simulink model "ACA_ModelLegoCar_v071"  (R2017b)
settings: Solver=VariableStepAuto  StartTime=0.0  StopTime=20  RelTol=1e-20
PreLoadFcn:
  | InitPar7_1
values from neighbouring files (symbols this model uses):
  CM_Actuator_NonlinarityType = 0    [InitPar7_1.m]
  CM_Actuator_SpeedDependent_MaxGainSpeedOffset = .1    (= 0.1)    [InitPar7_1.m]
  CM_Actuator_SpeedDependent_MinGain = 0.5    [InitPar7_1.m]
  CM_Actuator_SpeedDependent_ZeroSpeedGain = 0.7    [InitPar7_1.m]
  CM_CarWaight = 2    [InitPar7_1.m]
  CM_EnableActuatorQuantizer = 1    [InitPar7_1.m]
  CM_EnableBlockWheel = 1    [InitPar7_1.m]
  CM_EnableWheelSpin = 1    [InitPar7_1.m]
  CM_PWM_FixedOff_offset = 25    [InitPar7_1.m]
  CM_PWM_Type = 1    [InitPar7_1.m]
  CM_RelativeTorqueConstant = 0.0023    [InitPar7_1.m]
  CM_ViscousFriction = 0.018    [InitPar7_1.m]
  CM_WheelInertia = 0.000009    (= 9e-06)    [InitPar7_1.m]
  CM_WheelRadius = 0.03    [InitPar7_1.m]
  CM_WheelSpinInputSlope = 84.5    [InitPar7_1.m]
  CM_WheelSpinInputThresholdStandStill = 70    [InitPar7_1.m]
  FWS_EnableSensor = 0    [InitPar7_1.m]
  GravitinationalAcceleration = 9.82    [InitPar7_1.m]
  MAS_EnablePeriodicErrorAmplitude = 1    [InitPar7_1.m]
  MAS_EnableSensorQuantizer = 1    [InitPar7_1.m]
  MAS_PeriodicErrorAmplitude = 0.7*2*pi/360    (= 0.012217304764)    [InitPar7_1.m]
  One = 1    [InitPar7_1.m]
  Rad2DegFactor = 360/2/pi    (= 57.2957795131)    [InitPar7_1.m]
  USS_EnableError = 1    [InitPar7_1.m]
  USS_EnableSensorQuantizer = 1    [InitPar7_1.m]
  USS_LargeMaxValue = 1    [InitPar7_1.m]
  USS_UnitConversion = 1    [InitPar7_1.m]
libraries: simulink x3
settings Model: Creator=au521529  LastModifiedBy=au521529

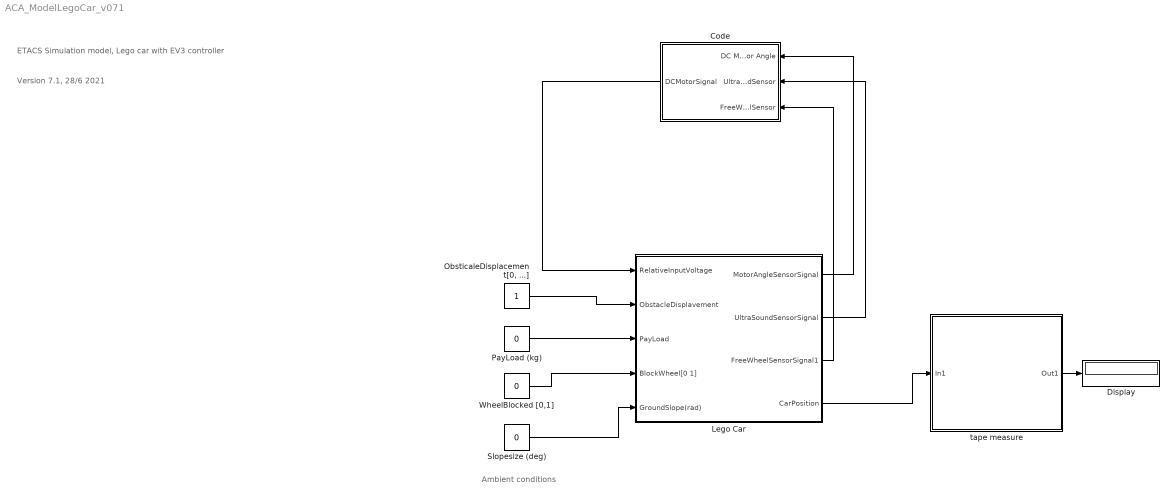
== system ACA_ModelLegoCar_v071 ==
  note: Ambient conditions
  note: Version 7.1, 28/6 2021
  note: ETACS Simulation model, Lego car with EV3 controller
  Code : Subsystem
      mask Display: image('Pic_SimulinkController.jpg');
  Display : Display
      settings: Decimation=2
  Lego Car : Subsystem
      mask DialogControl DescGroupVar Prompt: Logo Car
      mask DialogControl DescTextVar Prompt: This block simulates the mechanical part of the Lego Car. The imput is the scaled DC motor voltage [-100;0;100], where "100" corresponds to the maximum voltage, and "0" corresponds to 0 V. The Lego car has a base waight, driving the no-load dynamics. An additional payload can be applied by teh input port PayLoad (additional waigth in kg).
      mask Display: image(imread('FotoLegoBil.jpg'))
  "ObsticaleDisplacement[0, ...]" : Constant
  PayLoad (kg) : Constant  Value=0
  Slopesize (deg) : Constant  Value=0
  WheelBlocked [0,1] : Constant  Value=0
  tape measure : Subsystem
      mask Display: image('Pic_MaaleBaand.jpg');
  wires:
  Lego Car/1(MotorAngleSensorSignal) -> Code/1(DC Motor Angle)
  Lego Car/2(UltraSoundSensorSignal) -> Code/2(UltraSoundSensor)
  Lego Car/4(CarPosition) -> tape measure/1(In1)
  tape measure/1(Out1) -> Display/1
  Code/1(DCMotorSignal) -> Lego Car/1(RelativeInputVoltage)
  "ObsticaleDisplacement[0, ...]"/1 -> Lego Car/2("ObstacleDisplavement ")
  PayLoad (kg)/1 -> Lego Car/3(PayLoad)
  WheelBlocked [0,1]/1 -> Lego Car/4(BlockWheel[0 1])
  Lego Car/3(FreeWheelSensorSignal1) -> Code/3(FreeWheelSensor)
  Slopesize (deg)/1 -> Lego Car/5(GroundSlope(rad))

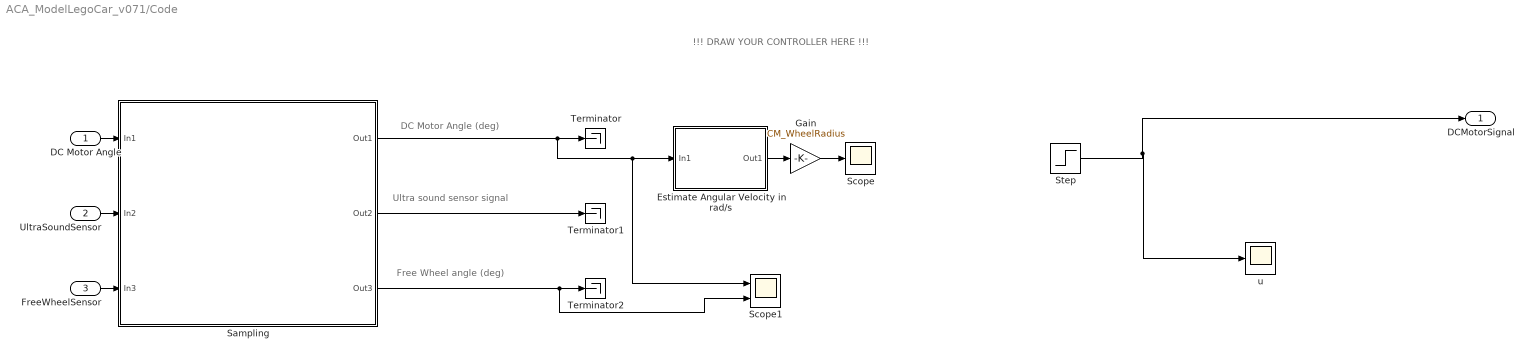
== system ACA_ModelLegoCar_v071/Code ==
  note: Ultra sound sensor signal
  note: Free Wheel angle (deg)
  note: DC Motor Angle (deg)
  note: !!! DRAW YOUR CONTROLLER HERE !!!
  DC Motor Angle : Inport
  UltraSoundSensor : Inport  Port=2
  FreeWheelSensor : Inport  Port=3
  Estimate Angular Velocity in rad/s : Subsystem
  Gain : Gain  Gain=CM_WheelRadius
  Sampling : Subsystem  mask{SystemTs=.01}
      mask prompts: SystemTs "Sampling time in seconds"
      mask DialogControl SystemTs Tooltip: Enter sampling time in seconds
      mask Display: image('Pic_Sampling.jpg');
  Scope : Scope
  Scope1 : Scope  NumInputPorts=2
  Step : Step  After=50  SampleTime=0
  Terminator : Terminator
  Terminator1 : Terminator
  Terminator2 : Terminator
  u : Scope
  DCMotorSignal : Outport
  wires:
  DC Motor Angle/1 -> Sampling/1(In1)
  UltraSoundSensor/1 -> Sampling/2(In2)
  Sampling/1(Out1) -> Scope1/1, Estimate Angular Velocity in rad/s/1(In1), Terminator/1
  Sampling/2(Out2) -> Terminator1/1
  Step/1 -> DCMotorSignal/1, u/1
  Estimate Angular Velocity in rad/s/1(Out1) -> Gain/1
  FreeWheelSensor/1 -> Sampling/3(In3)
  Sampling/3(Out3) -> Scope1/2, Terminator2/1
  Gain/1 -> Scope/1

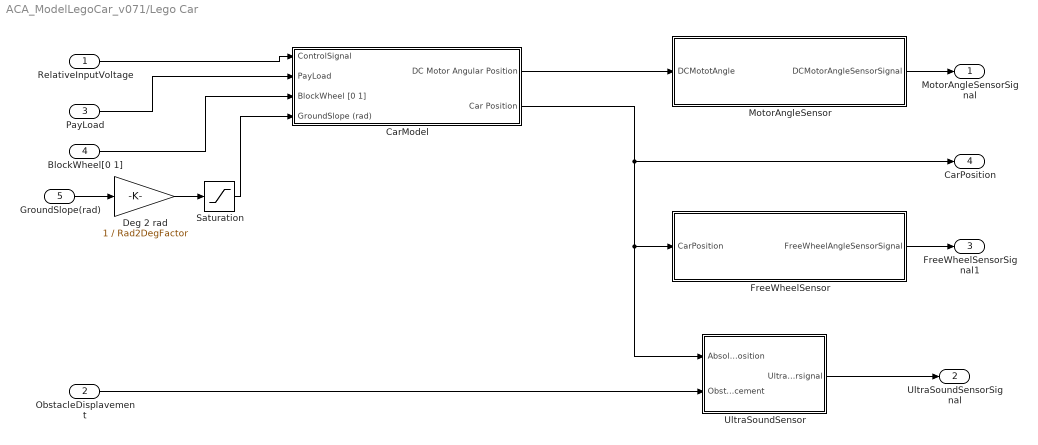
== system ACA_ModelLegoCar_v071/Lego Car ==
  RelativeInputVoltage : Inport
  "ObstacleDisplavement " : Inport  Port=2
  PayLoad : Inport  Port=3
  BlockWheel[0 1] : Inport  Port=4
  GroundSlope(rad) : Inport  Port=5
  CarModel : Subsystem
  Deg 2 rad : Gain  Gain=1 / Rad2DegFactor
  FreeWheelSensor : Subsystem
  MotorAngleSensor : Subsystem
  Saturation : Saturate  UpperLimit=pi/2*.99  LowerLimit=-pi/2*.99
  UltraSoundSensor : Subsystem
  MotorAngleSensorSignal : Outport
  UltraSoundSensorSignal : Outport  Port=2
  FreeWheelSensorSignal1 : Outport  Port=3
  CarPosition : Outport  Port=4
  wires:
  RelativeInputVoltage/1 -> CarModel/1(ControlSignal)
  "ObstacleDisplavement "/1 -> UltraSoundSensor/2(ObstacleDisplacement)
  UltraSoundSensor/1(UltraSoundSensorsignal) -> UltraSoundSensorSignal/1
  MotorAngleSensor/1(DCMotorAngleSensorSignal) -> MotorAngleSensorSignal/1
  CarModel/1(DC Motor Angular Position) -> MotorAngleSensor/1(DCMototAngle)
  PayLoad/1 -> CarModel/2(PayLoad)
  BlockWheel[0 1]/1 -> CarModel/3(BlockWheel [0 1])
  CarModel/2(Car Position) -> FreeWheelSensor/1(CarPosition), UltraSoundSensor/1(AbsoluteCarPosition), CarPosition/1
  FreeWheelSensor/1(FreeWheelAngleSensorSignal) -> FreeWheelSensorSignal1/1
  GroundSlope(rad)/1 -> Deg 2 rad/1
  Deg 2 rad/1 -> Saturation/1
  Saturation/1 -> CarModel/4(GroundSlope (rad))

== system ACA_ModelLegoCar_v071/tape measure ==
  In1 : Inport
  Gain : Gain  Gain=100
  Out1 : Outport
  wires:
  In1/1 -> Gain/1
  Gain/1 -> Out1/1

== system ACA_ModelLegoCar_v071/Code/Estimate Angular Velocity in rad//s ==
  In1 : Inport
  1/Ts : Gain  Gain=1/.01
  Sum : Sum  Inputs=|+-
  Unit Delay : UnitDelay  SampleTime=-1
  deg2rad : Gain  Gain=2*pi/360
  Out1 : Outport
  wires:
  Unit Delay/1 -> Sum/2
  In1/1 -> deg2rad/1
  deg2rad/1 -> Unit Delay/1, Sum/1
  1/Ts/1 -> Out1/1
  Sum/1 -> 1/Ts/1

== system ACA_ModelLegoCar_v071/Code/Sampling ==
  note: !!! DRAW YOUR CONTROLLER HERE !!!
  In1 : Inport
  In2 : Inport  Port=2
  In3 : Inport  Port=3
  Zero-Order Hold1 : ZeroOrderHold  SampleTime=SystemTs
  Zero-Order Hold2 : ZeroOrderHold  SampleTime=SystemTs
  Zero-Order Hold3 : ZeroOrderHold  SampleTime=SystemTs
  Out1 : Outport
  Out2 : Outport  Port=2
  Out3 : Outport  Port=3
  wires:
  In1/1 -> Zero-Order Hold2/1
  In2/1 -> Zero-Order Hold1/1
  Zero-Order Hold1/1 -> Out2/1
  Zero-Order Hold2/1 -> Out1/1
  Zero-Order Hold3/1 -> Out3/1
  In3/1 -> Zero-Order Hold3/1

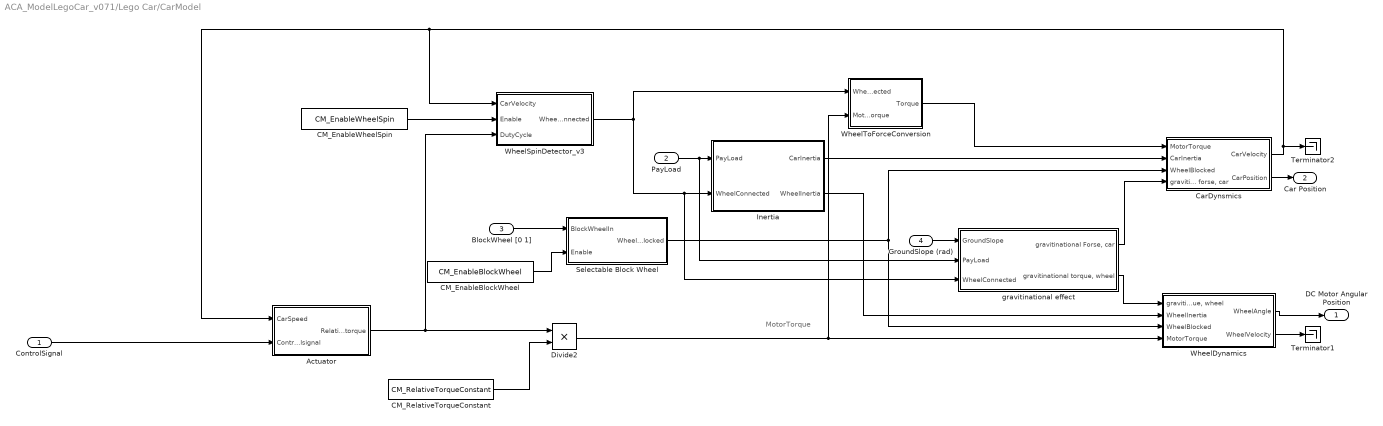
== system ACA_ModelLegoCar_v071/Lego Car/CarModel ==
  note: MotorTorque
  ControlSignal : Inport
  PayLoad : Inport  Port=2
  BlockWheel [0 1] : Inport  Port=3
  GroundSlope (rad) : Inport  Port=4
  Actuator : Subsystem
  CM_EnableBlockWheel : Constant  Value=CM_EnableBlockWheel
  CM_EnableWheelSpin : Constant  Value=CM_EnableWheelSpin
  CM_RelativeTorqueConstant : Constant  Value=CM_RelativeTorqueConstant
  CarDynsmics : Subsystem
  Divide2 : Product  Inputs=**
  Inertia : Subsystem
  Selectable Block Wheel : Subsystem
  Terminator1 : Terminator
  Terminator2 : Terminator
  WheelDynamics : Subsystem
  WheelSpinDetector_v3 : Subsystem
  WheelToForceConversion : Subsystem
  gravitinational effect : Subsystem
  DC Motor Angular Position : Outport
  Car Position : Outport  Port=2
  wires:
  Divide2/1 -> WheelToForceConversion/2(MotorTorque), WheelDynamics/4(MotorTorque)
  CM_RelativeTorqueConstant/1 -> Divide2/2
  PayLoad/1 -> gravitinational effect/2(PayLoad), Inertia/1(PayLoad)
  CM_EnableBlockWheel/1 -> Selectable Block Wheel/2(Enable)
  BlockWheel [0 1]/1 -> Selectable Block Wheel/1(BlockWheelIn)
  CM_EnableWheelSpin/1 -> WheelSpinDetector_v3/2(Enable)
  WheelToForceConversion/1(Torque) -> CarDynsmics/1(MotorTorque)
  Inertia/1(CarInertia) -> CarDynsmics/2(CarInertia)
  CarDynsmics/2(CarPosition) -> Car Position/1
  Inertia/2(WheelInertia) -> WheelDynamics/2(WheelInertia)
  WheelDynamics/1(WheelAngle) -> DC Motor Angular Position/1
  Selectable Block Wheel/1(WheelBlocked) -> WheelDynamics/3(WheelBlocked), CarDynsmics/3(WheelBlocked)
  WheelDynamics/2(WheelVelocity) -> Terminator1/1
  WheelSpinDetector_v3/1(WheelConnected) -> gravitinational effect/3(WheelConnected), Inertia/2(WheelConnected), WheelToForceConversion/1(WheelConnected)
  CarDynsmics/1(CarVelocity) -> Terminator2/1, Actuator/1(CarSpeed), WheelSpinDetector_v3/1(CarVelocity)
  Actuator/1(Relativetorque) -> Divide2/1, WheelSpinDetector_v3/3(DutyCycle)
  ControlSignal/1 -> Actuator/2(Controlsignal)
  gravitinational effect/2("gravitinational torque, wheel") -> WheelDynamics/1("gravitinational torque, wheel")
  gravitinational effect/1("gravitinational Forse, car") -> CarDynsmics/4("gravitinational forse, car")
  GroundSlope (rad)/1 -> gravitinational effect/1(GroundSlope)

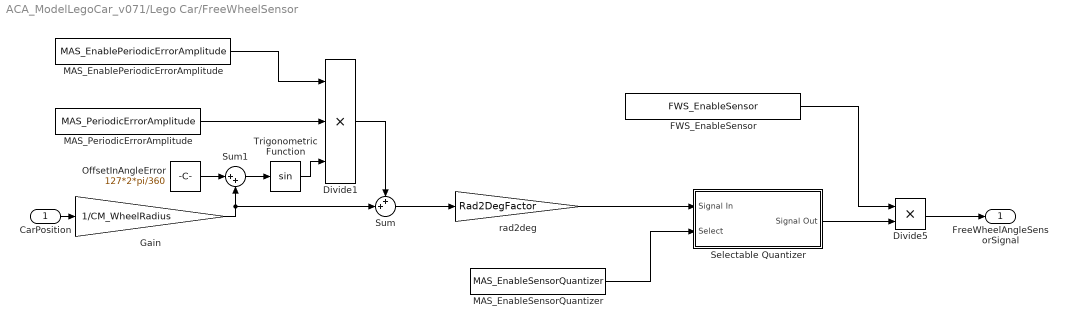
== system ACA_ModelLegoCar_v071/Lego Car/FreeWheelSensor ==
  CarPosition : Inport
  Divide1 : Product  Inputs=***
  Divide5 : Product  Inputs=**
  FWS_EnableSensor : Constant  Value=FWS_EnableSensor
  Gain : Gain  Gain=1/CM_WheelRadius
  MAS_EnablePeriodicErrorAmplitude : Constant  Value=MAS_EnablePeriodicErrorAmplitude
  MAS_EnableSensorQuantizer : Constant  Value=MAS_EnableSensorQuantizer
  MAS_PeriodicErrorAmplitude : Constant  Value=MAS_PeriodicErrorAmplitude
  OffsetInAngleError : Constant  Value=127*2*pi/360
  Selectable Quantizer : Subsystem
  Sum : Sum  Inputs=++|
  Sum1 : Sum  Inputs=|++
  Trigonometric Function : Trigonometry
  rad2deg : Gain  Gain=Rad2DegFactor
  FreeWheelAngleSensorSignal : Outport
  wires:
  Divide1/1 -> Sum/1
  Sum/1 -> rad2deg/1
  rad2deg/1 -> Selectable Quantizer/1(Signal In)
  MAS_EnableSensorQuantizer/1 -> Selectable Quantizer/2(Select)
  Trigonometric Function/1 -> Divide1/3
  MAS_PeriodicErrorAmplitude/1 -> Divide1/2
  MAS_EnablePeriodicErrorAmplitude/1 -> Divide1/1
  Sum1/1 -> Trigonometric Function/1
  OffsetInAngleError/1 -> Sum1/1
  Gain/1 -> Sum/2, Sum1/2
  CarPosition/1 -> Gain/1
  Selectable Quantizer/1(Signal Out) -> Divide5/2
  Divide5/1 -> FreeWheelAngleSensorSignal/1
  FWS_EnableSensor/1 -> Divide5/1

== system ACA_ModelLegoCar_v071/Lego Car/MotorAngleSensor ==
  DCMototAngle : Inport
  Divide1 : Product  Inputs=***
  MAS_EnablePeriodicErrorAmplitude : Constant  Value=MAS_EnablePeriodicErrorAmplitude
  MAS_EnableSensorQuantizer : Constant  Value=MAS_EnableSensorQuantizer
  MAS_PeriodicErrorAmplitude : Constant  Value=MAS_PeriodicErrorAmplitude
  Selectable Quantizer : Subsystem
  Sum : Sum  Inputs=++|
  Trigonometric Function : Trigonometry
  rad2deg : Gain  Gain=Rad2DegFactor
  DCMotorAngleSensorSignal : Outport
  wires:
  Divide1/1 -> Sum/1
  DCMototAngle/1 -> Trigonometric Function/1, Sum/2
  Sum/1 -> rad2deg/1
  rad2deg/1 -> Selectable Quantizer/1(Signal In)
  MAS_EnableSensorQuantizer/1 -> Selectable Quantizer/2(Select)
  Trigonometric Function/1 -> Divide1/3
  MAS_PeriodicErrorAmplitude/1 -> Divide1/2
  MAS_EnablePeriodicErrorAmplitude/1 -> Divide1/1
  Selectable Quantizer/1(Signal Out) -> DCMotorAngleSensorSignal/1

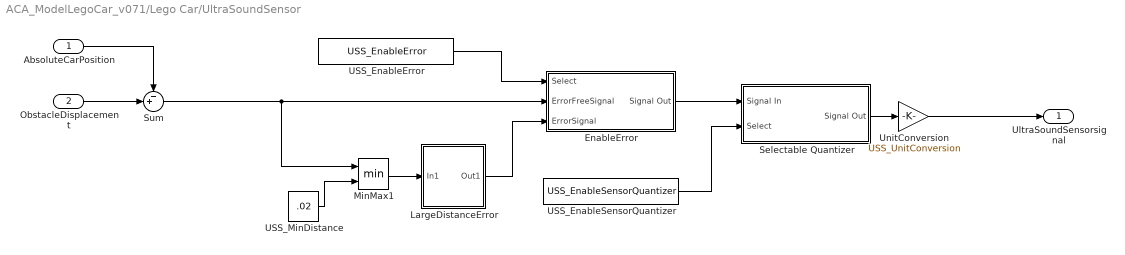
== system ACA_ModelLegoCar_v071/Lego Car/UltraSoundSensor ==
  AbsoluteCarPosition : Inport
  ObstacleDisplacement : Inport  Port=2
  EnableError : Subsystem
  LargeDistanceError : Subsystem
  MinMax1 : MinMax  Inputs=2
  Selectable Quantizer : Subsystem
  Sum : Sum  Inputs=-+|
  USS_EnableError : Constant  Value=USS_EnableError
  USS_EnableSensorQuantizer : Constant  Value=USS_EnableSensorQuantizer
  USS_MinDistance : Constant  Value=.02
  UnitConversion : Gain  Gain=USS_UnitConversion
  UltraSoundSensorsignal : Outport
  wires:
  ObstacleDisplacement/1 -> Sum/2
  AbsoluteCarPosition/1 -> Sum/1
  USS_MinDistance/1 -> MinMax1/2
  Sum/1 -> EnableError/2(ErrorFreeSignal), MinMax1/1
  LargeDistanceError/1(Out1) -> EnableError/3(ErrorSignal)
  MinMax1/1 -> LargeDistanceError/1(In1)
  Selectable Quantizer/1(Signal Out) -> UnitConversion/1
  USS_EnableSensorQuantizer/1 -> Selectable Quantizer/2(Select)
  EnableError/1(Signal Out) -> Selectable Quantizer/1(Signal In)
  USS_EnableError/1 -> EnableError/1(Select)
  UnitConversion/1 -> UltraSoundSensorsignal/1

== system ACA_ModelLegoCar_v071/Lego Car/CarModel/Actuator ==
  note: Duty sycle
  CarSpeed : Inport
  Controlsignal : Inport  Port=2
  ActuatorNonlinarity : Subsystem
  CM_Actuator_NonlinarityType : Constant  Value=CM_Actuator_NonlinarityType
  CM_PWM_Type : Constant  Value=CM_PWM_Type
  CM_RelativeTorqueConstant1 : Constant  Value=CM_EnableActuatorQuantizer
  PWM and communication : Subsystem
  Relativetorque : Outport
  wires:
  PWM and communication/1(DutyScycle(procentage)) -> ActuatorNonlinarity/2(ControlSignal)
  CM_RelativeTorqueConstant1/1 -> PWM and communication/2(EnableQuantizer)
  CM_Actuator_NonlinarityType/1 -> ActuatorNonlinarity/3(NonlinarityType [0 1])
  CM_PWM_Type/1 -> PWM and communication/3(Select_PWM_type)
  ActuatorNonlinarity/1(DutyScycle(procentage)) -> Relativetorque/1
  Controlsignal/1 -> PWM and communication/1(ControlSignal)
  CarSpeed/1 -> ActuatorNonlinarity/1(CarSpeed)

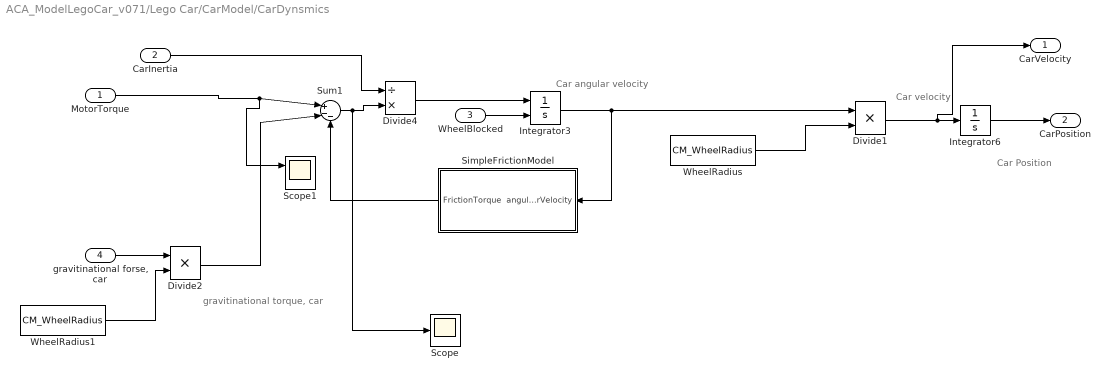
== system ACA_ModelLegoCar_v071/Lego Car/CarModel/CarDynsmics ==
  note: gravitinational torque, car
  note: Car velocity
  note: Car angular velocity
  note: Car Position
  MotorTorque : Inport
  CarInertia : Inport  Port=2
  WheelBlocked : Inport  Port=3
  "gravitinational forse, car" : Inport  Port=4
  Divide1 : Product  Inputs=**
  Divide2 : Product  Inputs=**
  Divide4 : Product  Inputs=/*
  Integrator3 : Integrator  ExternalReset=level
  Integrator6 : Integrator
  Scope : Scope
  Scope1 : Scope  NumInputPorts=2
  SimpleFrictionModel : Subsystem
  Sum1 : Sum  Inputs=|+--
  WheelRadius : Constant  Value=CM_WheelRadius
  WheelRadius1 : Constant  Value=CM_WheelRadius
  CarVelocity : Outport
  CarPosition : Outport  Port=2
  wires:
  Divide4/1 -> Integrator3/1
  Sum1/1 -> Scope/1, Divide4/2
  Integrator3/1 -> Divide1/1, SimpleFrictionModel/1(angularVelocity)
  Integrator6/1 -> CarPosition/1
  WheelBlocked/1 -> Integrator3/2
  SimpleFrictionModel/1(FrictionTorque) -> Sum1/3
  Divide1/1 -> CarVelocity/1, Integrator6/1
  WheelRadius/1 -> Divide1/2
  "gravitinational forse, car"/1 -> Divide2/1
  WheelRadius1/1 -> Divide2/2
  MotorTorque/1 -> Scope1/1, Sum1/1
  CarInertia/1 -> Divide4/1
  Divide2/1 -> Sum1/2

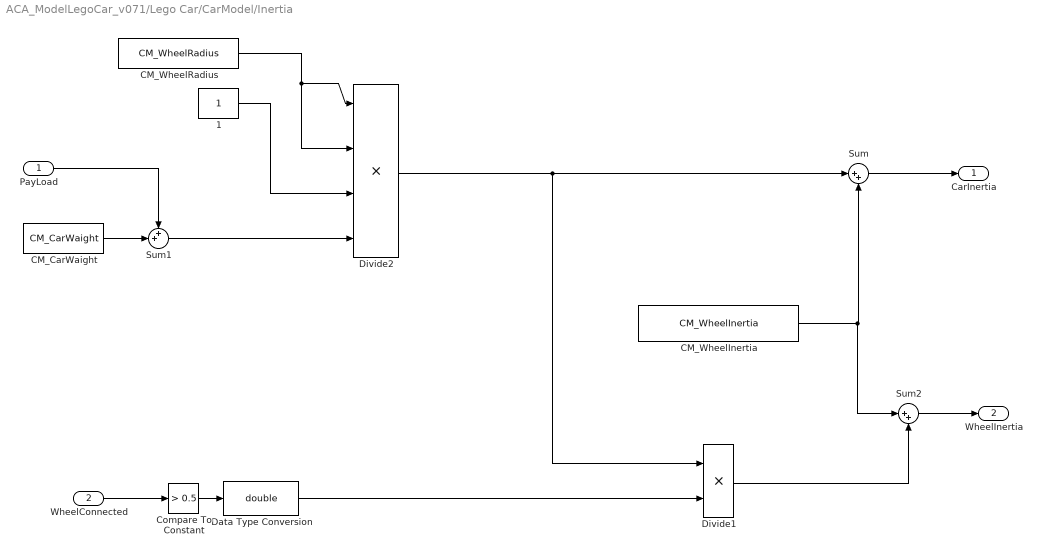
== system ACA_ModelLegoCar_v071/Lego Car/CarModel/Inertia ==
  PayLoad : Inport
  WheelConnected : Inport  Port=2
  "1 " : Constant
  CM_CarWaight : Constant  Value=CM_CarWaight
  CM_WheelInertia : Constant  Value=CM_WheelInertia
  CM_WheelRadius : Constant  Value=CM_WheelRadius
  Compare To Constant : simulink/Logic and Bit Operations/Compare To Constant  relop=>  const=0.5  OutDataTypeStr=boolean
  Data Type Conversion : DataTypeConversion  OutDataTypeStr=double
  Divide1 : Product  Inputs=**
  Divide2 : Product  Inputs=****
  Sum : Sum  Inputs=|++
  Sum1 : Sum  Inputs=++|
  Sum2 : Sum  Inputs=|++
  CarInertia : Outport
  WheelInertia : Outport  Port=2
  wires:
  CM_WheelRadius/1 -> Divide2/1, Divide2/2
  PayLoad/1 -> Sum1/1
  "1 "/1 -> Divide2/3
  CM_CarWaight/1 -> Sum1/2
  Sum1/1 -> Divide2/4
  Divide2/1 -> Divide1/1, Sum/1
  Sum/1 -> CarInertia/1
  CM_WheelInertia/1 -> Sum2/1, Sum/2
  Data Type Conversion/1 -> Divide1/2
  Compare To Constant/1 -> Data Type Conversion/1
  WheelConnected/1 -> Compare To Constant/1
  Divide1/1 -> Sum2/2
  Sum2/1 -> WheelInertia/1

== system ACA_ModelLegoCar_v071/Lego Car/CarModel/Selectable Block Wheel ==
  BlockWheelIn : Inport
  Enable : Inport  Port=2
  Compare To Constant : simulink/Logic and Bit Operations/Compare To Constant  relop=>  const=0.5  OutDataTypeStr=boolean
  Data Type Conversion : DataTypeConversion  OutDataTypeStr=double
  Divide4 : Product  Inputs=**
  WheelBlocked : Outport
  wires:
  Divide4/1 -> WheelBlocked/1
  Enable/1 -> Divide4/2
  Compare To Constant/1 -> Data Type Conversion/1
  Data Type Conversion/1 -> Divide4/1
  BlockWheelIn/1 -> Compare To Constant/1

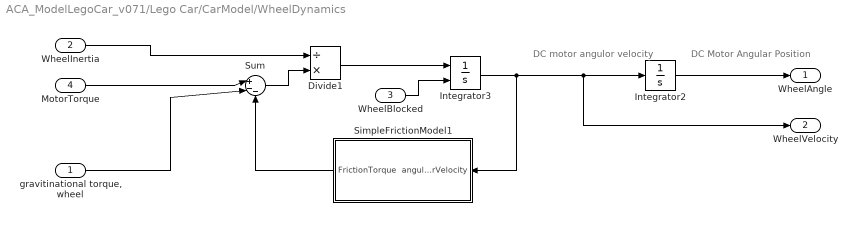
== system ACA_ModelLegoCar_v071/Lego Car/CarModel/WheelDynamics ==
  note: DC Motor Angular Position
  note: DC motor angulor velocity
  "gravitinational torque, wheel" : Inport
  WheelInertia : Inport  Port=2
  WheelBlocked : Inport  Port=3
  MotorTorque : Inport  Port=4
  Divide1 : Product  Inputs=/*
  Integrator2 : Integrator
  Integrator3 : Integrator  ExternalReset=level
  SimpleFrictionModel1 : Subsystem
  Sum : Sum  Inputs=|+--
  WheelAngle : Outport
  WheelVelocity : Outport  Port=2
  wires:
  Integrator2/1 -> WheelAngle/1
  Sum/1 -> Divide1/2
  WheelInertia/1 -> Divide1/1
  MotorTorque/1 -> Sum/1
  Integrator3/1 -> WheelVelocity/1, Integrator2/1, SimpleFrictionModel1/1(angularVelocity)
  Divide1/1 -> Integrator3/1
  WheelBlocked/1 -> Integrator3/2
  SimpleFrictionModel1/1(FrictionTorque) -> Sum/3
  "gravitinational torque, wheel"/1 -> Sum/2

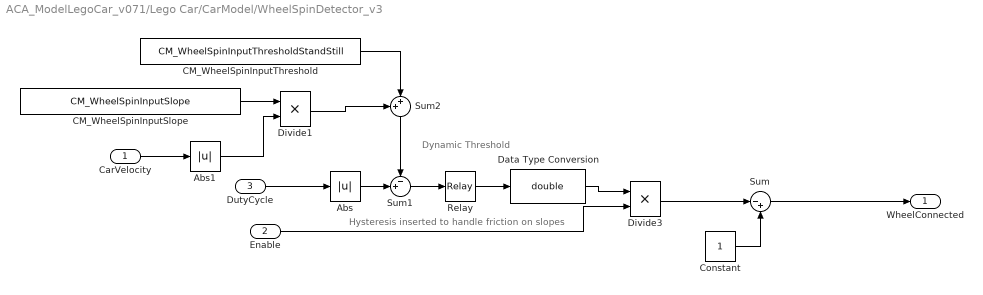
== system ACA_ModelLegoCar_v071/Lego Car/CarModel/WheelSpinDetector_v3 ==
  note: Hysteresis inserted to handle friction on slopes
  note: Dynamic Threshold
  CarVelocity : Inport
  Enable : Inport  Port=2
  DutyCycle : Inport  Port=3
  Abs : Abs
  Abs1 : Abs
  CM_WheelSpinInputSlope : Constant  Value=CM_WheelSpinInputSlope
  CM_WheelSpinInputThreshold : Constant  Value=CM_WheelSpinInputThresholdStandStill
  Constant : Constant
  Data Type Conversion : DataTypeConversion  OutDataTypeStr=double
  Divide1 : Product  Inputs=**
  Divide3 : Product  Inputs=**
  Relay : Relay  OnSwitchValue=.01  OffSwitchValue=.001
  Sum : Sum  Inputs=|-+
  Sum1 : Sum  Inputs=-+|
  Sum2 : Sum  Inputs=++|
  WheelConnected : Outport
  wires:
  Data Type Conversion/1 -> Divide3/1
  Relay/1 -> Data Type Conversion/1
  DutyCycle/1 -> Abs/1
  Enable/1 -> Divide3/2
  Constant/1 -> Sum/2
  Divide3/1 -> Sum/1
  Abs/1 -> Sum1/2
  Sum1/1 -> Relay/1
  CM_WheelSpinInputThreshold/1 -> Sum2/2
  Sum2/1 -> Sum1/1
  Divide1/1 -> Sum2/1
  CM_WheelSpinInputSlope/1 -> Divide1/1
  CarVelocity/1 -> Abs1/1
  Abs1/1 -> Divide1/2
  Sum/1 -> WheelConnected/1

== system ACA_ModelLegoCar_v071/Lego Car/CarModel/WheelToForceConversion ==
  WheelConnected : Inport
  MotorTorque : Inport  Port=2
  1 : Constant
  Divide6 : Product  Inputs=***
  Scope : Scope
  Torque : Outport
  wires:
  WheelConnected/1 -> Divide6/2
  1/1 -> Divide6/1
  Divide6/1 -> Scope/1, Torque/1
  MotorTorque/1 -> Divide6/3

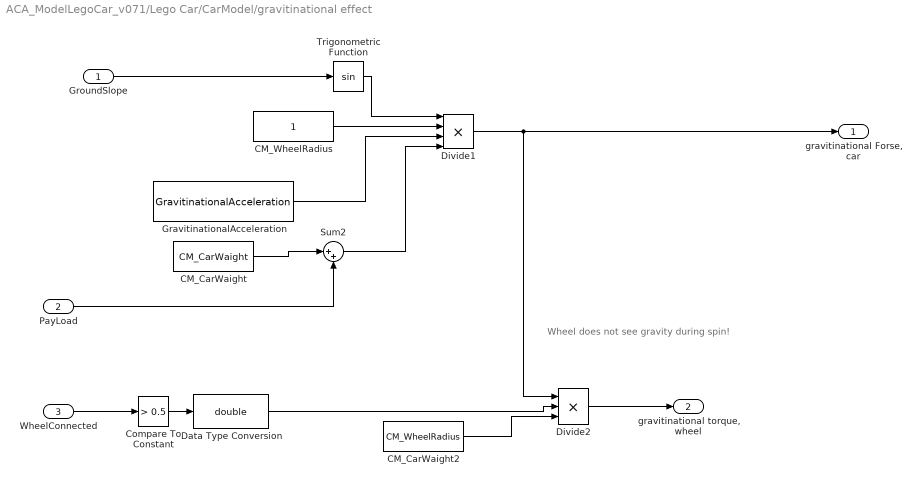
== system ACA_ModelLegoCar_v071/Lego Car/CarModel/gravitinational effect ==
  note: Wheel does not see gravity during spin!
  GroundSlope : Inport
  PayLoad : Inport  Port=2
  WheelConnected : Inport  Port=3
  CM_CarWaight : Constant  Value=CM_CarWaight
  CM_CarWaight2 : Constant  Value=CM_WheelRadius
  "CM_WheelRadius " : Constant
  Compare To Constant : simulink/Logic and Bit Operations/Compare To Constant  relop=>  const=0.5  OutDataTypeStr=boolean
  Data Type Conversion : DataTypeConversion  OutDataTypeStr=double
  Divide1 : Product  Inputs=****
  Divide2 : Product  Inputs=***
  GravitinationalAcceleration : Constant  Value=GravitinationalAcceleration
  Sum2 : Sum  Inputs=|++
  Trigonometric Function : Trigonometry
  "gravitinational Forse, car" : Outport
  "gravitinational torque, wheel" : Outport  Port=2
  wires:
  PayLoad/1 -> Sum2/2
  Trigonometric Function/1 -> Divide1/1
  Sum2/1 -> Divide1/4
  "CM_WheelRadius "/1 -> Divide1/2
  GravitinationalAcceleration/1 -> Divide1/3
  CM_CarWaight/1 -> Sum2/1
  GroundSlope/1 -> Trigonometric Function/1
  WheelConnected/1 -> Compare To Constant/1
  Compare To Constant/1 -> Data Type Conversion/1
  Data Type Conversion/1 -> Divide2/2
  Divide2/1 -> "gravitinational torque, wheel"/1
  CM_CarWaight2/1 -> Divide2/3
  Divide1/1 -> "gravitinational Forse, car"/1, Divide2/1

== system ACA_ModelLegoCar_v071/Lego Car/FreeWheelSensor/Selectable Quantizer ==
  Signal In : Inport
  Select : Inport  Port=2
  Divide4 : Product  Inputs=**
  Divide5 : Product  Inputs=**
  One : Constant
  Quantizer : Quantizer  QuantizationInterval=1
  Sum1 : Sum  Inputs=-+|
  Sum2 : Sum  Inputs=+|+
  Signal Out : Outport
  wires:
  Sum2/1 -> Signal Out/1
  Quantizer/1 -> Divide5/1
  Signal In/1 -> Divide4/2, Quantizer/1
  Sum1/1 -> Divide4/1
  Select/1 -> Sum1/1, Divide5/2
  Divide4/1 -> Sum2/2
  One/1 -> Sum1/2
  Divide5/1 -> Sum2/1

== system ACA_ModelLegoCar_v071/Lego Car/MotorAngleSensor/Selectable Quantizer ==
  Signal In : Inport
  Select : Inport  Port=2
  Divide4 : Product  Inputs=**
  Divide5 : Product  Inputs=**
  One : Constant
  Quantizer : Quantizer  QuantizationInterval=1
  Sum1 : Sum  Inputs=-+|
  Sum2 : Sum  Inputs=+|+
  Signal Out : Outport
  wires:
  Sum2/1 -> Signal Out/1
  Quantizer/1 -> Divide5/1
  Signal In/1 -> Divide4/2, Quantizer/1
  Sum1/1 -> Divide4/1
  Select/1 -> Sum1/1, Divide5/2
  Divide4/1 -> Sum2/2
  One/1 -> Sum1/2
  Divide5/1 -> Sum2/1

== system ACA_ModelLegoCar_v071/Lego Car/UltraSoundSensor/EnableError ==
  Select : Inport
  ErrorFreeSignal : Inport  Port=2
  ErrorSignal : Inport  Port=3
  Divide4 : Product  Inputs=**
  Divide5 : Product  Inputs=**
  One : Constant  Value=One
  Sum1 : Sum  Inputs=-+|
  Sum2 : Sum  Inputs=+|+
  Signal Out : Outport
  wires:
  Sum2/1 -> Signal Out/1
  ErrorSignal/1 -> Divide5/1
  Sum1/1 -> Divide4/1
  Select/1 -> Sum1/1, Divide5/2
  Divide4/1 -> Sum2/2
  One/1 -> Sum1/2
  Divide5/1 -> Sum2/1
  ErrorFreeSignal/1 -> Divide4/2

== system ACA_ModelLegoCar_v071/Lego Car/UltraSoundSensor/LargeDistanceError ==
  In1 : Inport
  1 : Constant
  Divide : Product  Inputs=/*
  Divide1 : Product  Inputs=**
  Gain : Gain  Gain=-1
  Math Function : Math  SaturateOnIntegerOverflow=on
  MinMax1 : MinMax  Inputs=2
  Sum1 : Sum  Inputs=-+|
  USS_LargeErrorSlope : Constant  Value=.7
  USS_LargeMaxValue : Constant  Value=USS_LargeMaxValue
  Out1 : Outport
  wires:
  Math Function/1 -> Sum1/1
  Sum1/1 -> Divide1/1
  USS_LargeMaxValue/1 -> Divide1/2
  Gain/1 -> Divide/1
  USS_LargeErrorSlope/1 -> Gain/1
  Divide/1 -> Math Function/1
  In1/1 -> MinMax1/2, Divide/2
  1/1 -> Sum1/2
  Divide1/1 -> MinMax1/1
  MinMax1/1 -> Out1/1

== system ACA_ModelLegoCar_v071/Lego Car/UltraSoundSensor/Selectable Quantizer ==
  Signal In : Inport
  Select : Inport  Port=2
  Divide4 : Product  Inputs=**
  Divide5 : Product  Inputs=**
  One : Constant
  Quantizer : Quantizer  QuantizationInterval=1
  Sum1 : Sum  Inputs=-+|
  Sum2 : Sum  Inputs=+|+
  Signal Out : Outport
  wires:
  Sum2/1 -> Signal Out/1
  Quantizer/1 -> Divide5/1
  Signal In/1 -> Divide4/2, Quantizer/1
  Sum1/1 -> Divide4/1
  Select/1 -> Sum1/1, Divide5/2
  Divide4/1 -> Sum2/2
  One/1 -> Sum1/2
  Divide5/1 -> Sum2/1

== system ACA_ModelLegoCar_v071/Lego Car/CarModel/Actuator/ActuatorNonlinarity ==
  note: Constant period PWM
  CarSpeed : Inport
  ControlSignal : Inport  Port=2
  NonlinarityType [0 1] : Inport  Port=3
  Abs1 : Abs
  Divide3 : Product  Inputs=**
  Index Vector : MultiPortSwitch  DataPortOrder=Zero-based contiguous  Inputs=2
  Saturation : Saturate  UpperLimit=1  LowerLimit=0
  Tytpe 1: Polonium : Subsystem
  DutyScycle(procentage) : Outport
  wires:
  ControlSignal/1 -> Divide3/1, Index Vector/2
  Saturation/1 -> Index Vector/1
  Index Vector/1 -> DutyScycle(procentage)/1
  NonlinarityType [0 1]/1 -> Saturation/1
  CarSpeed/1 -> Abs1/1
  Divide3/1 -> Index Vector/3
  Abs1/1 -> Tytpe 1: Polonium/1(In1)
  Tytpe 1: Polonium/1(Out1) -> Divide3/2

== system ACA_ModelLegoCar_v071/Lego Car/CarModel/Actuator/PWM and communication ==
  ControlSignal : Inport
  EnableQuantizer : Inport  Port=2
  Select_PWM_type : Inport  Port=3
  PWM : Subsystem
  Saturation : Saturate  UpperLimit=100  LowerLimit=-100
  Selectable Quantizer : Subsystem
  DutyScycle(procentage) : Outport
  wires:
  ControlSignal/1 -> Saturation/1
  EnableQuantizer/1 -> Selectable Quantizer/2(Enable)
  Select_PWM_type/1 -> PWM/2(PWM_ Type [1 2])
  Selectable Quantizer/1(Signal Out) -> PWM/1(ControlSignal)
  PWM/1(DutyScycle(procentage)) -> DutyScycle(procentage)/1
  Saturation/1 -> Selectable Quantizer/1(Signal In)

== system ACA_ModelLegoCar_v071/Lego Car/CarModel/CarDynsmics/SimpleFrictionModel ==
  angularVelocity : Inport
  CM_ViscousFriction : Constant  Value=CM_ViscousFriction
  Divide4 : Product  Inputs=**
  FrictionTorque : Outport
  wires:
  angularVelocity/1 -> Divide4/2
  CM_ViscousFriction/1 -> Divide4/1
  Divide4/1 -> FrictionTorque/1

== system ACA_ModelLegoCar_v071/Lego Car/CarModel/WheelDynamics/SimpleFrictionModel1 ==
  angularVelocity : Inport
  CM_ViscousFriction : Constant  Value=CM_ViscousFriction
  Divide4 : Product  Inputs=**
  FrictionTorque : Outport
  wires:
  angularVelocity/1 -> Divide4/2
  CM_ViscousFriction/1 -> Divide4/1
  Divide4/1 -> FrictionTorque/1

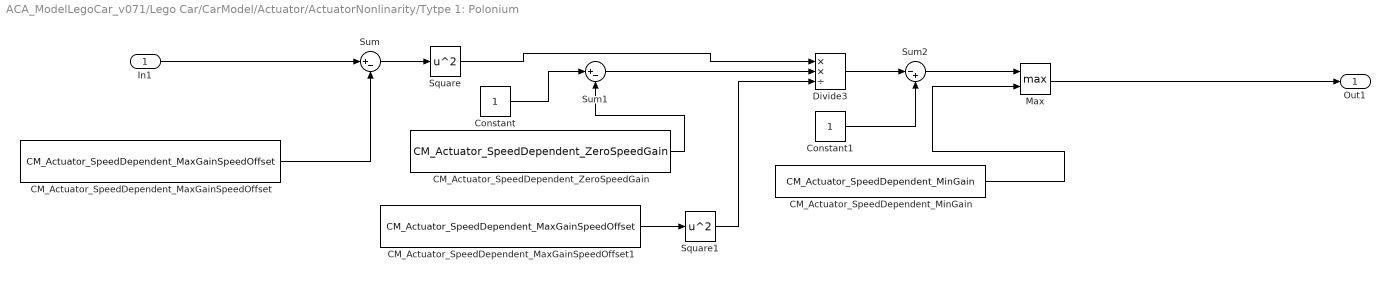
== system ACA_ModelLegoCar_v071/Lego Car/CarModel/Actuator/ActuatorNonlinarity/Tytpe 1: Polonium ==
  In1 : Inport
  CM_Actuator_SpeedDependent_MaxGainSpeedOffset : Constant  Value=CM_Actuator_SpeedDependent_MaxGainSpeedOffset
  CM_Actuator_SpeedDependent_MaxGainSpeedOffset1 : Constant  Value=CM_Actuator_SpeedDependent_MaxGainSpeedOffset
  CM_Actuator_SpeedDependent_MinGain : Constant  Value=CM_Actuator_SpeedDependent_MinGain
  CM_Actuator_SpeedDependent_ZeroSpeedGain : Constant  Value=CM_Actuator_SpeedDependent_ZeroSpeedGain
  Constant : Constant
  Constant1 : Constant
  Divide3 : Product  Inputs=**/
  Max : MinMax  Function=max  Inputs=2
  Square : Math  Operator=square  RndMeth=Zero  SaturateOnIntegerOverflow=on
  Square1 : Math  Operator=square  RndMeth=Zero  SaturateOnIntegerOverflow=on
  Sum : Sum  Inputs=|+-
  Sum1 : Sum  Inputs=|+-
  Sum2 : Sum  Inputs=|-+
  Out1 : Outport
  wires:
  In1/1 -> Sum/1
  Sum/1 -> Square/1
  CM_Actuator_SpeedDependent_MaxGainSpeedOffset/1 -> Sum/2
  Square1/1 -> Divide3/3
  Constant1/1 -> Sum2/2
  Constant/1 -> Sum1/1
  Sum2/1 -> Max/1
  Max/1 -> Out1/1
  Square/1 -> Divide3/1
  Sum1/1 -> Divide3/2
  Divide3/1 -> Sum2/1
  CM_Actuator_SpeedDependent_ZeroSpeedGain/1 -> Sum1/2
  CM_Actuator_SpeedDependent_MaxGainSpeedOffset1/1 -> Square1/1
  CM_Actuator_SpeedDependent_MinGain/1 -> Max/2

== system ACA_ModelLegoCar_v071/Lego Car/CarModel/Actuator/PWM and communication/PWM ==
  note: Constant period PWM
  ControlSignal : Inport
  PWM_ Type [1 2] : Inport  Port=2
  Abs1 : Abs
  CM_PWM_FixedOff_offset : Constant  Value=CM_PWM_FixedOff_offset
  Divide3 : Product  Inputs=*/
  Gain : Gain  Gain=100
  Index Vector : MultiPortSwitch  Inputs=2
  Saturation : Saturate  UpperLimit=3  LowerLimit=1
  Saturation1 : Saturate  UpperLimit=100  LowerLimit=-100
  Sum : Sum  Inputs=|++
  DutyScycle(procentage) : Outport
  wires:
  Saturation1/1 -> Abs1/1, Divide3/1, Index Vector/2
  Saturation/1 -> Index Vector/1
  Index Vector/1 -> DutyScycle(procentage)/1
  PWM_ Type [1 2]/1 -> Saturation/1
  ControlSignal/1 -> Saturation1/1
  Abs1/1 -> Sum/1
  Sum/1 -> Divide3/2
  CM_PWM_FixedOff_offset/1 -> Sum/2
  Divide3/1 -> Gain/1
  Gain/1 -> Index Vector/3

== system ACA_ModelLegoCar_v071/Lego Car/CarModel/Actuator/PWM and communication/Selectable Quantizer ==
  Signal In : Inport
  Enable : Inport  Port=2
  Divide4 : Product  Inputs=**
  Divide5 : Product  Inputs=**
  One : Constant
  Quantizer : Quantizer  QuantizationInterval=1
  Sum1 : Sum  Inputs=-+|
  Sum2 : Sum  Inputs=+|+
  Signal Out : Outport
  wires:
  Sum2/1 -> Signal Out/1
  Quantizer/1 -> Divide5/1
  Signal In/1 -> Divide4/2, Quantizer/1
  Sum1/1 -> Divide4/1
  Enable/1 -> Sum1/1, Divide5/2
  Divide4/1 -> Sum2/2
  One/1 -> Sum1/2
  Divide5/1 -> Sum2/1
